simulink model "fl"  (R2022b)
settings: Solver=VariableStepAuto  StartTime=0.0  StopTime=3  RelTol=1e-3
values from neighbouring files (symbols this model uses):
  I_m = [params.permanent.J/params.physical.mu0*params.permanent.l(1) ... (first row only)    [pole_placement.m]
  K_xyz = place(A_xyz,B_xyz,[-0.5,-0.5,-0.5,-40,-30,-2000,-2000,-9000,-25,-20])    [pole_placement.m]
  params =     [Dataset.mat]
  x0 = [0.001 -0.003 0.0765018943706 0.628318530718 0 0 0 0 0 0 0 0]    [Dataset.mat]    (also in convergence_plot_func.m = xLp + [x,y,z, zeros(1,9)]')
  xLp = [0 0 0.0365018943706 0 0 0 0 0 0 0 0 0]    [Dataset.mat]
settings Model: Creator=pal12  LastModifiedBy=pal12
settings SolverCC: ZeroCrossAlgorithm=Adaptive
settings DebuggingCC: IgnoredZcDiagnostic=none

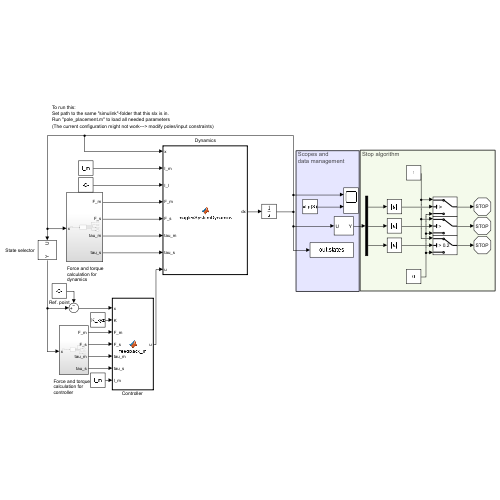
[thumbnail: Simulink's stored preview of the top-level diagram]
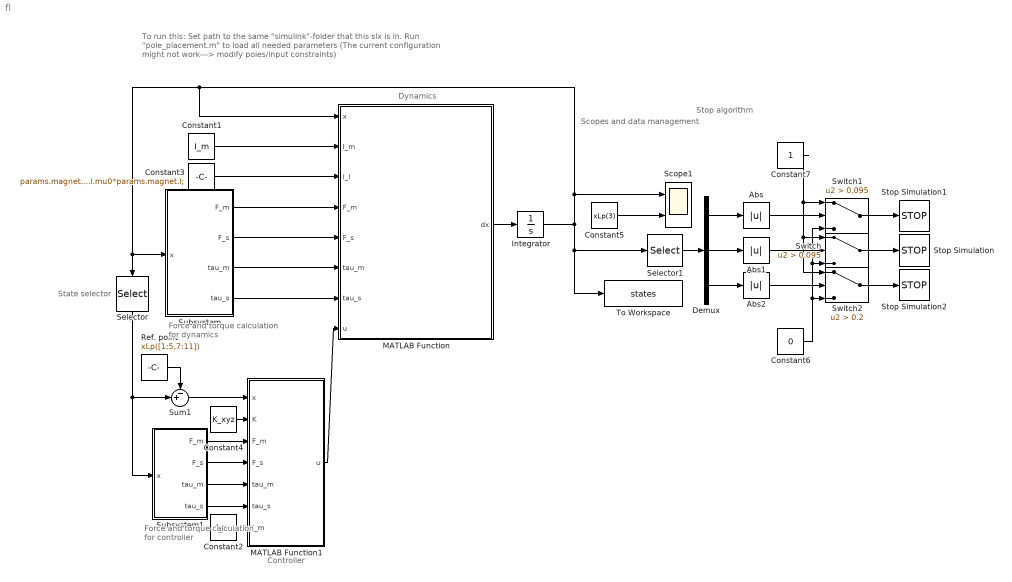
== system fl ==
  note: Scopes and
      | data management
  note: Controller
  note: State selector
  note: Force and torque calculation for dynamics
  note: Stop algorithm
  note: Dynamics
  note: Force and torque calculation for controller
  note: To run this:
      | Set path to the same "simulink"-folder that this slx is in.
      | Run "pole_placement.m" to load all needed parameters
      | (The current configuration might not work---> modify poles/input constraints)
  Abs : Abs  SaturateOnIntegerOverflow=off
  Abs1 : Abs  SaturateOnIntegerOverflow=off
  Abs2 : Abs  SaturateOnIntegerOverflow=off
  Constant1 : Constant  Value=I_m
  Constant2 : Constant  Value=I_m
  Constant3 : Constant  Value=params.magnet.J/params.physical.mu0*params.magnet.l;
  Constant4 : Constant  Value=K_xyz
  Constant5 : Constant  Value=xLp(3)
  Constant6 : Constant  Value=0
  Constant7 : Constant
  Demux : Demux  Outputs=3
  Integrator : Integrator  InitialCondition=x0
  MATLAB Function : MATLAB Function  TreatAsAtomicUnit=on
  MATLAB Function1 : MATLAB Function  TreatAsAtomicUnit=on
  Ref. point : Constant  Value=xLp([1:5,7:11])
  Scope1 : Scope  NumInputPorts=2
  Selector : Selector  InputPortWidth=12  IndexOptions=Index vector (dialog)  Indices=[1 2 3 4 5 7 8 9 10 11]  OutputSizes=1
  Selector1 : Selector  InputPortWidth=12  IndexOptions=Index vector (dialog)  Indices=[1 2 3]  OutputSizes=1
  Stop Simulation : Stop
  Stop Simulation1 : Stop
  Stop Simulation2 : Stop
  Subsystem : Subsystem
  Subsystem1 : Subsystem
  Sum1 : Sum  Inputs=-+|
  Switch : Switch  Criteria=u2 > Threshold  Threshold=0.095  SaturateOnIntegerOverflow=off  InputSameDT=off
  Switch1 : Switch  Criteria=u2 > Threshold  Threshold=0.095  SaturateOnIntegerOverflow=off  InputSameDT=off
  Switch2 : Switch  Criteria=u2 > Threshold  Threshold=0.2  SaturateOnIntegerOverflow=off  InputSameDT=off
  To Workspace : ToWorkspace  VariableName=states  SampleTime=-1
      settings: Save2DSignal=2-D array (concatenate along first dimension)
  wires:
  MATLAB Function/1(dx) -> Integrator/1
  Constant1/1 -> MATLAB Function/2(I_m)
  Integrator/1 -> MATLAB Function/1(x), Selector/1, Subsystem/1(x), Scope1/1, To Workspace/1, Selector1/1
  Subsystem/1(F_m) -> MATLAB Function/4(F_m)
  Subsystem/2(F_s) -> MATLAB Function/5(F_s)
  Subsystem/3(tau_m) -> MATLAB Function/6(tau_m)
  Subsystem/4(tau_s) -> MATLAB Function/7(tau_s)
  Constant3/1 -> MATLAB Function/3(I_l)
  Subsystem1/1(F_m) -> MATLAB Function1/3(F_m)
  Subsystem1/2(F_s) -> MATLAB Function1/4(F_s)
  Constant2/1 -> MATLAB Function1/7(I_m)
  Constant4/1 -> MATLAB Function1/2(K)
  Sum1/1 -> MATLAB Function1/1(x)
  Subsystem1/3(tau_m) -> MATLAB Function1/5(tau_m)
  Subsystem1/4(tau_s) -> MATLAB Function1/6(tau_s)
  Switch/1 -> Stop Simulation/1
  Selector1/1 -> Demux/1
  Switch1/1 -> Stop Simulation1/1
  Abs/1 -> Switch1/2
  Demux/1 -> Abs/1
  Demux/2 -> Abs1/1
  Demux/3 -> Abs2/1
  Switch2/1 -> Stop Simulation2/1
  Abs1/1 -> Switch/2
  Abs2/1 -> Switch2/2
  Constant6/1 -> Switch1/3, Switch/3, Switch2/3
  Constant7/1 -> Switch1/1, Switch/1, Switch2/1
  Constant5/1 -> Scope1/2
  Ref. point/1 -> Sum1/1
  Selector/1 -> Subsystem1/1(x), Sum1/2
  MATLAB Function1/1(u) -> MATLAB Function/8(u)

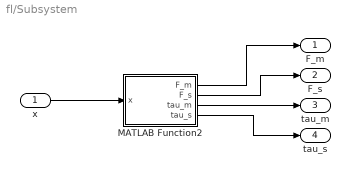
== system fl/Subsystem ==
  x : Inport
  MATLAB Function2 : MATLAB Function  TreatAsAtomicUnit=on
  F_m : Outport
  F_s : Outport  Port=2
  tau_m : Outport  Port=3
  tau_s : Outport  Port=4
  wires:
  MATLAB Function2/2(F_s) -> F_s/1
  MATLAB Function2/1(F_m) -> F_m/1
  x/1 -> MATLAB Function2/1(x)
  MATLAB Function2/3(tau_m) -> tau_m/1
  MATLAB Function2/4(tau_s) -> tau_s/1

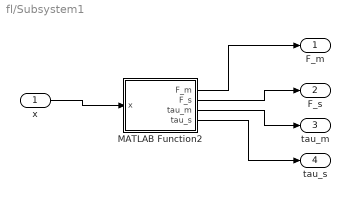
== system fl/Subsystem1 ==
  x : Inport
  MATLAB Function2 : MATLAB Function  TreatAsAtomicUnit=on
  F_m : Outport
  F_s : Outport  Port=2
  tau_m : Outport  Port=3
  tau_s : Outport  Port=4
  wires:
  MATLAB Function2/2(F_s) -> F_s/1
  MATLAB Function2/1(F_m) -> F_m/1
  x/1 -> MATLAB Function2/1(x)
  MATLAB Function2/3(tau_m) -> tau_m/1
  MATLAB Function2/4(tau_s) -> tau_s/1

== matlab function fl/MATLAB Function1 ==
  data: x input; K input; u output; params parameter; F_m input; F_s input; tau_m input; tau_s input; I_m input
function u = feedback_ln(x, K, params, F_m, F_s,tau_m,tau_s, I_m)
    lim = 5;
    g = [
    params.magnet.m*eye(3), zeros(3);
    zeros(3), diag(params.magnet.I)
    ];

    %h = [zeros(3,1); cross(x(10:12),diag(params.magnet.I)*x(10:12))]-[zeros(2,1);params.physical.g;zeros(3,1)];
    h = [zeros(6,1)]-[zeros(2,1);params.physical.g;zeros(3,1)];
    
    Fm = [F_m;tau_m];
    Fs = [F_s;tau_s];

    u_nonlin=(h(1:5)-Fm(1:5,:)*I_m);
    u = Fs(1:5,:)\(u_nonlin.*1-g(1:5,1:6)*K*x);
    
    for i=1:4
        if u(i) < -lim
            u(i) = -lim;
        elseif u(i) > lim
            u(i) = lim;
        end
    end



    
    %u = Fs(1:3,:)\(h(1:3)-Fm(1:3,:)*I_m-g(1:3,1:6)*K*x([1:3,6:8]));

== matlab function fl/MATLAB Function ==
  data: x input; I_m input; I_l input; params parameter; F_m input; F_s input; tau_m input; tau_s input; u input; dx output
function dx  = maglevSystemDynamics(x,I_m,I_l,params,F_m,F_s,tau_m,tau_s,u)
    %{
    Computes the derivative of the state for a magnetic levitation system.
    - x: current state
    - u: control input
    - params: system parameters
    %}

    F = F_m*I_m+F_s*u;
    tau = tau_m*I_m+tau_s*u;
    
    % Setting up system matrices
    A = [
        zeros(6), eye(6);
        zeros(6), zeros(6)
        ];

    B = [
        zeros(6);
        eye(6)
        ];
    
    % Mass and inertia properties of the magnet
    M = [
        params.magnet.m*eye(3), zeros(3);
        zeros(3), diag(params.magnet.I)
        ];
    
    % Computing the nonlinear function f(x,u)
    f = M\([F;tau]-[zeros(3,1); cross(x(10:12),diag(params.magnet.I)*x(10:12))])-[zeros(2,1);params.physical.g;zeros(3,1)];
    
    dx = A*x+B*f;

%     B1 = B_m(:,1:3).*I_l;
%     B2 = B_m(:,4:6).*I_m(1)+B_m(:,7:9).*I_m(2)+B_m(:,10:12).*I_m(3)+B_m(:,13:15).*I_m(4);
%     B3 = B_m(:,16:18).*u(1)+B_m(:,19:21).*u(2)+B_m(:,22:24).*u(3)+B_m(:,25:27).*u(4);
%     B_temp = B1+B2+B3;
%     y = B_temp(:);
end

== matlab function fl/Subsystem/MATLAB Function2 ==
  data: F_m output; F_s output; tau_m output; tau_s output; x input; params parameter
function [F_m,F_s,tau_m,tau_s] = fcn(x,params)
[F_m,F_s,tau_m,tau_s] = computeForceAndTorque_sim(x,0,params,"fast");
%     Bm = zeros(3, length(params.sensors.x));
%     Bm_m = zeros(3, length(params.sensors.x)*4);
%     Bm_s = zeros(3, length(params.sensors.x)*4);
% 
%     % Field from levitating magnet
%     I = params.magnet.J/params.physical.mu0*params.magnet.l;
% 
%     [phiLocal,rhoLocal,zLocal] = c2p(params.sensors.x-x(1),params.sensors.y-x(2),params.sensors.z-x(3));
%     BpolLocal = field(phiLocal,rhoLocal,zLocal, ...
%         params.magnet.r,params.magnet.l, ...
%         params.physical.mu0, ...
%         1);
% 
%     [bx,by,bz] = p2c(BpolLocal(1,:),BpolLocal(2,:),BpolLocal(3,:));
% 
%     Bm = Bm + [bx;by;bz];
% 
%     % Field from permanent magnets
%     for i = 1:length(params.permanent.r)
% 
%         [phiLocal,rhoLocal,zLocal] = c2p(params.sensors.x-params.permanent.x(i),params.sensors.y-params.permanent.y(i),params.sensors.z-params.permanent.z(i));
%         BpolLocal = field(phiLocal,rhoLocal,zLocal, ...
%             params.permanent.r(i),params.permanent.l(i), ...
%             params.physical.mu0, ...
%             1);
% 
%         [bx,by,bz] = p2c(BpolLocal(1,:),BpolLocal(2,:),BpolLocal(3,:));
% 
%         Bm_m(:,1+(i-1)*length(params.sensors.x):i*length(params.sensors.x)) = [bx;by;bz];
%     end
% 
%     % Field from solenoids
%     for i = 1:length(params.solenoids.r)
%         [phiLocal,rhoLocal,zLocal] = c2p(params.sensors.x-params.solenoids.x(i),params.sensors.y-params.solenoids.y(i),params.sensors.z-params.solenoids.z(i));
%         
%         BpolLocal = field(phiLocal,rhoLocal,zLocal,...
%             params.solenoids.r(i),params.solenoids.l(i), ...
%             params.physical.mu0, ...
%             params.solenoids.nw);
% 
%         [bx,by,bz] = p2c(BpolLocal(1,:),BpolLocal(2,:),BpolLocal(3,:));
% 
%         Bm_s(:,1+(i-1)*length(params.sensors.x):i*length(params.sensors.x)) = [bx;by;bz];
%     end
%     
%     Bs = [Bm Bm_m Bm_s];
end

== matlab function fl/Subsystem1/MATLAB Function2 ==
  data: F_m output; F_s output; x input; params parameter; tau_m output; tau_s output
function [F_m,F_s,tau_m,tau_s] = fcn(x,params)
[F_m,F_s,tau_m,tau_s] = computeForceAndTorque(x,0,params,"fast");
